simulink model "Simulink1"  (Simulink 5.0)
settings: Solver=ode45  StartTime=0.0  StopTime=50.0  RelTol=1e-5
settings Model: LastModifiedBy=stevel

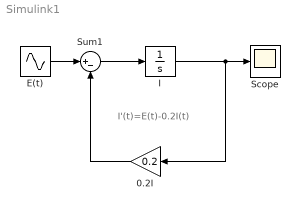
== system Simulink1 ==
  note: I'(t)=E(t)-0.2I(t)
  0.2I : Gain  Orientation=left  Gain=0.2  SaturateOnIntegerOverflow=on
  E(t) : Sin  Amplitude=5  SampleTime=0
  I : Integrator
  Scope : Scope
  Sum1 : Sum  Inputs=|+-  SaturateOnIntegerOverflow=on
  wires:
  E(t)/1 -> Sum1/1
  Sum1/1 -> I/1
  I/1 -> Scope/1, 0.2I/1
  0.2I/1 -> Sum1/2
